simulink model "FireFighter_original"  (R2014a)
settings: Solver=ode45  StartTime=0.0  StopTime=150  RelTol=1e-3
undefined symbols (not defined in the file): DiscIntNeverNeededParam, sigbuilder_block
libraries: simulink x68
(part 6 of 6)

== system FireFighter_original/FF_Signals4/Inaccuracy2/Subsystem2/FireFighter ==
  note: current speed
  note: speed=90
  pos : Inport
  Constant : Constant  Value=0
  Constant1 : Constant  Value=0
  Constant2 : Constant  Value=0
  Discrete Derivative : simulink/Discrete/Discrete Derivative  gainval=1.0  ICPrevScaledInput=0.0  InputProcessing=Inherited  OutMin=[]  OutMax=[]  OutDataType=fixdt(1, 16)  OutScaling=2^-10  DoSatur=off
  Discrete PID Controller : simulink/Continuous/PID Controller  Controller=PI  TimeDomain=Discrete-time  SampleTime=-1  IntegratorMethod=Forward Euler  FilterMethod=Forward Euler  Form=Parallel  P=0.05  I=0.000228325  D=0  N=100  InitialConditionSource=internal  InitialConditionForIntegrator=0  InitialConditionForFilter=0  ExternalReset=none  LimitOutput=on  UpperSaturationLimit=1  LowerSaturationLimit=-1  LinearizeAsGain=off  AntiWindupMode=back-calculation  Kb=0.01  TrackingMode=off  Kt=1  PParamMin=[]  PParamMax=[]  IParamMin=[]  IParamMax=[]  DParamMin=[]  DParamMax=[]  NParamMin=[]  NParamMax=[]  KbParamMin=[]  KbParamMax=[]  KtParamMin=[]  KtParamMax=[]  POutMin=[]  POutMax=[]  IOutMin=[]  IOutMax=[]  DOutMin=[]  DOutMax=[]  NOutMin=[]  NOutMax=[]  KbOutMin=[]  KbOutMax=[]  KtOutMin=[]  KtOutMax=[]  IntegratorOutMin=[]  IntegratorOutMax=[]  FilterOutMin=[]  FilterOutMax=[]  SumOutMin=[]  SumOutMax=[]  SumI1OutMin=[]  SumI1OutMax=[]  SumI2OutMin=[]  SumI2OutMax=[]  SumI3OutMin=[]  SumI3OutMax=[]  SumDOutMin=[]  SumDOutMax=[]  SaturationOutMin=[]  SaturationOutMax=[]  IntegratorContinuousStateAttributes=''  IntegratorStateMustResolveToSignalObject=off  IntegratorRTWStateStorageClass=Auto  FilterContinuousStateAttributes=''  FilterStateMustResolveToSignalObject=off  FilterRTWStateStorageClass=Auto
  Discrete PID Controller1 : simulink/Continuous/PID Controller  Controller=PI  TimeDomain=Discrete-time  SampleTime=-1  IntegratorMethod=Forward Euler  FilterMethod=Forward Euler  Form=Parallel  P=0.05  I=0.000228325  D=0  N=100  InitialConditionSource=internal  InitialConditionForIntegrator=0  InitialConditionForFilter=0  ExternalReset=none  LimitOutput=on  UpperSaturationLimit=1  LowerSaturationLimit=-1  LinearizeAsGain=off  AntiWindupMode=back-calculation  Kb=0.01  TrackingMode=off  Kt=1  PParamMin=[]  PParamMax=[]  IParamMin=[]  IParamMax=[]  DParamMin=[]  DParamMax=[]  NParamMin=[]  NParamMax=[]  KbParamMin=[]  KbParamMax=[]  KtParamMin=[]  KtParamMax=[]  POutMin=[]  POutMax=[]  IOutMin=[]  IOutMax=[]  DOutMin=[]  DOutMax=[]  NOutMin=[]  NOutMax=[]  KbOutMin=[]  KbOutMax=[]  KtOutMin=[]  KtOutMax=[]  IntegratorOutMin=[]  IntegratorOutMax=[]  FilterOutMin=[]  FilterOutMax=[]  SumOutMin=[]  SumOutMax=[]  SumI1OutMin=[]  SumI1OutMax=[]  SumI2OutMin=[]  SumI2OutMax=[]  SumI3OutMin=[]  SumI3OutMax=[]  SumDOutMin=[]  SumDOutMax=[]  SaturationOutMin=[]  SaturationOutMax=[]  IntegratorContinuousStateAttributes=''  IntegratorStateMustResolveToSignalObject=off  IntegratorRTWStateStorageClass=Auto  FilterContinuousStateAttributes=''  FilterStateMustResolveToSignalObject=off  FilterRTWStateStorageClass=Auto
  Fast - to -Slow : RateTransition  OutPortSampleTimeMultiple=0.05  OutPortSampleTime=0.1
  Fast - to -Slow1 : RateTransition  OutPortSampleTimeMultiple=0.05  OutPortSampleTime=0.1
  Fast - to -Slow2 : RateTransition  OutPortSampleTimeMultiple=0.05  OutPortSampleTime=0.1
  Gain1 : Gain  Gain=-1
  Scope{1..2,4..9,11..13} (11 alike) : Scope
      Scope1 settings: YMin=-300  YMax=300  SaveName=ScopeData52
      Scope11 settings: YMin=-300  YMax=300  SaveName=ScopeData28
      Scope12 settings: YMin=-300  YMax=300  SaveName=ScopeData30
      Scope13 settings: SaveName=ScopeData31
      Scope2 settings: YMin=-300  YMax=300  SaveName=ScopeData2
      Scope4 settings: YMin=-300  YMax=300  SaveName=ScopeData17
      Scope5 settings: SaveName=ScopeData20
      Scope6 settings: YMin=-300  YMax=300  SaveName=ScopeData18
      Scope7 settings: YMin=-300  YMax=300  SaveName=ScopeData24
      Scope8 settings: TimeRange=10  SaveName=ScopeData25
      Scope9 settings: SaveName=ScopeData38
  Slow - to - Fast : RateTransition  OutPortSampleTimeMultiple=0.05  OutPortSampleTime=0.05
  Slow - to - Fast1 : RateTransition  OutPortSampleTimeMultiple=0.05  OutPortSampleTime=0.05
  Sum : Sum  Inputs=|+-
  Switch : Switch
  Switch1 : Switch
  gas : Outport
  brake : Outport  Port=2
  wires:
  Discrete Derivative/1 -> Scope8/1, Sum/2
  Discrete PID Controller/1 -> Scope2/1, Scope7/1, Switch/1, Switch/2, Switch1/2, Gain1/1
  Gain1/1 -> Switch1/3
  Switch/1 -> Slow - to - Fast/1, Scope4/1
  Constant/1 -> Switch/3, Switch1/1
  Switch1/1 -> Slow - to - Fast1/1, Scope6/1
  pos/1 -> Scope13/1, Fast - to -Slow/1
  Sum/1 -> Discrete PID Controller/1, Scope9/1
  Fast - to -Slow/1 -> Discrete Derivative/1, Scope5/1
  Slow - to - Fast/1 -> Scope11/1, gas/1
  Slow - to - Fast1/1 -> Scope12/1, brake/1
  Constant2/1 -> Fast - to -Slow1/1
  Fast - to -Slow1/1 -> Sum/1
  Discrete PID Controller1/1 -> Scope1/1
  Constant1/1 -> Fast - to -Slow2/1
  Fast - to -Slow2/1 -> Discrete PID Controller1/1

== stateflow chart FireFighter_original/Helicopter1 ==
  state FlyOn
    en:
    hold = 1;
    during:
    HFFPos = FFPos;
    HPos = HPos_In;
    inacc = FFPosInacc[1] - FFPosInacc[0];
    Signal_Reply_Out[0] =Signal_In[0];
    Signal_Reply_Out[1] =Signal_In[1];
    state srchID=getClosest [function]
      state [min,max] = getComposedInaccuracy(min1,max1, min2,max2) [function]
        state x_abs =abs(x) [function]
          (default) -> (junction 3808)
          (junction 3808) -> (junction 3809) [order 1] : [x < 0]
          (junction 3808) -> (junction 3810) [order 2] : {x_abs = x;}
          (junction 3809) -> (junction 3811) : {x_abs = -1*x;}
          (junction 3811) -> (junction 3810)
          (junction 3810) -> (junction 3812)
        (default) -> (junction 3780)
        (junction 3780) -> (junction 3785) : {val[0] = abs(min2 - min1);
            | val[1] = abs(max2 - min1);
            | val[2] = abs(min2 - max1);
            | val[3] = abs(max2 - max1);
            | min = val[0];
            | max = val[0];
            | j =1;}
        (junction 3781) -> (junction 3782) [order 1] : [min > val[j]]
        (junction 3785) -> (junction 3781) [order 1] : [j<4]
        (junction 3781) -> (junction 3783) [order 2]
        (junction 3782) -> (junction 3784) : {min = val[j];}
        (junction 3784) -> (junction 3783)
        (junction 3783) -> (junction 3786)
        (junction 3789) -> (junction 3785) : {j++;}
        (junction 3785) -> (junction 3788) [order 2]
        (junction 3786) -> (junction 3787) [order 1] : [max < val[j]]
        (junction 3787) -> (junction 3790) : {max = val[j];}
        (junction 3786) -> (junction 3789) [order 2]
        (junction 3790) -> (junction 3789)
      (default) -> (junction 3745)
      (junction 3745) -> (junction 3746) : {
          | [Min[0],Max[0]]=getComposedInaccuracy(FFPosInacc[0],FFPosInacc[1],FFPos,FFPos);
          | [Min[1],Max[1]]=getComposedInaccuracy(FFPosInacc[0],FFPosInacc[1],HsPosInacc[0],HsPosInacc[1]);
          | [Min[2],Max[2]]=getComposedInaccuracy(FFPosInacc[0],FFPosInacc[1],HsPosInacc[2],HsPosInacc[3]);
          | inacc_min = Min[0];
          | srchID = HID;
          | i =1;
          | }
      (junction 3736) -> (junction 3724) [order 1] : [inacc_min > Min[i]]
      (junction 3746) -> (junction 3736) [order 1] : [i<3]
      (junction 3736) -> (junction 3738) [order 2]
      (junction 3724) -> (junction 3732) : {inacc_min = Min[i]; srchID = OHIDs[i-1];}
      (junction 3738) -> (junction 3746) : {i++;}
      (junction 3746) -> (junction 3740) [order 2]
      (junction 3732) -> (junction 3738)
    state inaccFuture=getInacc(dt) [function]
      (default) -> (junction 3488)
      (junction 3488) -> (junction 3489) [order 1] : [true]
      (junction 3488) -> (junction 3490) [order 2]
      (junction 3489) -> (junction 3491) : {inaccFuture = dt*inacc;}
      (junction 3491) -> (junction 3490)
      (junction 3490) -> (junction 3492)
    state Mediate
      en:
      time_last =0;
      time_period = 0;
      time_val = temporalCount(sec);
      du:
      time_val = temporalCount(sec);
    state HsSignals [function]
      (default) -> (junction 3581)
      (junction 3581) -> (junction 3580) [order 1] : [(Signal_Reply_In[0] != Signal_Out || Signal_Reply_In[0] != Signal_Out) && time_period < (time_val - time_last)]
      (junction 3581) -> (junction 3583) [order 2]
      (junction 3580) -> (junction 3586) : {time_period = time_val - time_last;}
      (junction 3583) -> (junction 3582) [order 1] : [Signal_Reply_In[0] == Signal_Out &&Signal_Reply_In[1] == Signal_Out]
      (junction 3583) -> (junction 3584) [order 2]
      (junction 3582) -> (junction 3585) : {Signal_Out = time_val; time_last = Signal_Out; }
      (junction 3585) -> (junction 3584)
      (junction 3586) -> (junction 3585)
      (junction 3584) -> (junction 3587)
    state OrganizeSearch
      en:
      hold = 0;
      time_last =0;
      time_period = 0;
      time_val = temporalCount(sec);
      Signal_Out = time_val;
      SearchID = getClosest();
      du:
      HsSignals();
      SearchID = getClosest();
      time_val = temporalCount(sec);
      ex:
      hold = 1;
      state InitializedSearch
      state LeadSearch
      state OtherSearch
        du:
        Search_Out = SearchID;
        ex:
        Search_Out = 0;
      (default) -> InitializedSearch
      InitializedSearch -> LeadSearch [order 1] : [SearchID == HID]
      InitializedSearch -> OtherSearch [order 2] : [SearchID != HID]
      OtherSearch -> LeadSearch : [SearchID == HID]
      LeadSearch -> OtherSearch : [SearchID != HID]
    state ToldToSearch
      en: hold = 0;
      ex: hold = 1;
    state InitializedSystem
      en:
      hold = 0;
      HFFPos = 0;
      ex:
      hold = 1;
    InitializedSystem -> Mediate [order 1] : [MID == HID]
    Mediate -> InitializedSystem [order 2] : [MID != HID && MID !=0]
    OrganizeSearch -> Mediate [order 1] : [inacc <= 5000]
    Mediate -> OrganizeSearch [order 1] : [ inacc > 5000  ]
    InitializedSystem -> ToldToSearch [order 2] : [Search_In[0] == HID || Search_In[1] == HID]
    ToldToSearch -> InitializedSystem : [Search_In[0] != HID && Search_In[1] != HID]
    (default) -> InitializedSystem
    OrganizeSearch -> InitializedSystem [order 2] : [MID != HID && MID !=0]
    OrganizeSearch -> InitializedSystem [order 3] : [(inacc+getInacc(time_period))  > 10000]
  state FlyOff
  FlyOn -> FlyOff : [SWITCH==0]
  FlyOff -> FlyOn : [SWITCH==1]
  (default) -> FlyOff
  data: x function_input double; x_abs function_output double; min1 function_input double; max1 function_input double; min function_output double; max function_output double; val temporary double size=4; min2 function_input double; max2 function_input double; j local double; srchID function_output double; Max temporary double size=3; Min temporary double size=3; inacc1 temporary double size=2; i local double; inacc_min local double; inaccFuture function_output double; dt function_input double; HID output =1; FFPos input; HFFPos output; HPos output double =0; HPos_In input double; FFPosInacc input size=2; HsPosInacc input size=4; SWITCH input double; OHIDs input size=2; OHPoss input size=2; OHFFPos input size=2; Search_In input size=2; SearchID local double; Search_Loc local double; MID input; Signal_In input size=2; Signal_Out output; Search_Out output; time_val local double; Signal_Reply_Out output size=2; Signal_Reply_In input size=2; valFF local double; time_period local double; time_last local double; inacc local double; hold output double

== stateflow chart FireFighter_original/Helicopter2 ==
  state FlyOn
    en:
    hold = 1;
    during:
    HFFPos = FFPos;
    HPos = HPos_In;
    inacc = FFPosInacc[1] - FFPosInacc[0];
    Signal_Reply_Out[0] =Signal_In[0];
    Signal_Reply_Out[1] =Signal_In[1];
    state srchID=getClosest [function]
      state [min,max] = getComposedInaccuracy(min1,max1, min2,max2) [function]
        state x_abs =abs(x) [function]
          (default) -> (junction 3883)
          (junction 3883) -> (junction 3884) [order 1] : [x < 0]
          (junction 3883) -> (junction 3885) [order 2] : {x_abs = x;}
          (junction 3884) -> (junction 3886) : {x_abs = -1*x;}
          (junction 3886) -> (junction 3885)
          (junction 3885) -> (junction 3887)
        (default) -> (junction 3855)
        (junction 3855) -> (junction 3860) : {val[0] = abs(min2 - min1);
            | val[1] = abs(max2 - min1);
            | val[2] = abs(min2 - max1);
            | val[3] = abs(max2 - max1);
            | min = val[0];
            | max = val[0];
            | j =1;}
        (junction 3856) -> (junction 3857) [order 1] : [min > val[j]]
        (junction 3860) -> (junction 3856) [order 1] : [j<4]
        (junction 3856) -> (junction 3858) [order 2]
        (junction 3857) -> (junction 3859) : {min = val[j];}
        (junction 3859) -> (junction 3858)
        (junction 3858) -> (junction 3861)
        (junction 3864) -> (junction 3860) : {j++;}
        (junction 3860) -> (junction 3863) [order 2]
        (junction 3861) -> (junction 3862) [order 1] : [max < val[j]]
        (junction 3862) -> (junction 3865) : {max = val[j];}
        (junction 3861) -> (junction 3864) [order 2]
        (junction 3865) -> (junction 3864)
      (default) -> (junction 3830)
      (junction 3830) -> (junction 3833) : {
          | [Min[0],Max[0]]=getComposedInaccuracy(FFPosInacc[0],FFPosInacc[1],FFPos,FFPos);
          | [Min[1],Max[1]]=getComposedInaccuracy(FFPosInacc[0],FFPosInacc[1],HsPosInacc[0],HsPosInacc[1]);
          | [Min[2],Max[2]]=getComposedInaccuracy(FFPosInacc[0],FFPosInacc[1],HsPosInacc[2],HsPosInacc[3]);
          | inacc_min = Min[0];
          | srchID = HID;
          | i =1;
          | }
      (junction 3831) -> (junction 3832) [order 1] : [inacc_min > Min[i]]
      (junction 3833) -> (junction 3831) [order 1] : [i<3]
      (junction 3831) -> (junction 3834) [order 2]
      (junction 3832) -> (junction 3835) : {inacc_min = Min[i]; srchID = OHIDs[i-1];}
      (junction 3834) -> (junction 3833) : {i++;}
      (junction 3833) -> (junction 3836) [order 2]
      (junction 3835) -> (junction 3834)
    state inaccFuture=getInacc(dt) [function]
      (default) -> (junction 3488)
      (junction 3488) -> (junction 3489) [order 1] : [true]
      (junction 3488) -> (junction 3490) [order 2]
      (junction 3489) -> (junction 3491) : {inaccFuture = dt*inacc;}
      (junction 3491) -> (junction 3490)
      (junction 3490) -> (junction 3492)
    state Mediate
      en:
      time_last =0;
      time_period = 0;
      time_val = temporalCount(sec);
      du:
      time_val = temporalCount(sec);
    state HsSignals [function]
      (default) -> (junction 3581)
      (junction 3581) -> (junction 3580) [order 1] : [(Signal_Reply_In[0] != Signal_Out || Signal_Reply_In[0] != Signal_Out) && time_period < (time_val - time_last)]
      (junction 3581) -> (junction 3583) [order 2]
      (junction 3580) -> (junction 3586) : {time_period = time_val - time_last;}
      (junction 3583) -> (junction 3582) [order 1] : [Signal_Reply_In[0] == Signal_Out &&Signal_Reply_In[1] == Signal_Out]
      (junction 3583) -> (junction 3584) [order 2]
      (junction 3582) -> (junction 3585) : {Signal_Out = time_val; time_last = Signal_Out; }
      (junction 3585) -> (junction 3584)
      (junction 3586) -> (junction 3585)
      (junction 3584) -> (junction 3587)
    state OrganizeSearch
      en:
      hold = 0;
      time_last =0;
      time_period = 0;
      time_val = temporalCount(sec);
      Signal_Out = time_val;
      SearchID = getClosest();
      du:
      HsSignals();
      SearchID = getClosest();
      time_val = temporalCount(sec);
      ex:
      hold = 1;
      state InitializeSearch
      state LeadSearch
      state OtherSearch
        du:
        Search_Out = SearchID;
        ex:
        Search_Out = 0;
      (default) -> InitializeSearch
      InitializeSearch -> LeadSearch [order 1] : [SearchID == HID]
      InitializeSearch -> OtherSearch [order 2] : [SearchID != HID]
      OtherSearch -> LeadSearch : [SearchID == HID]
      LeadSearch -> OtherSearch : [SearchID != HID]
    state ToldToSearch
      en: hold = 0;
      ex: hold = 1;
    state InitializedSystem
      en:
      hold = 0;
      HFFPos = 0;
      ex:
      hold = 1;
    InitializedSystem -> Mediate [order 1] : [MID == HID]
    Mediate -> InitializedSystem [order 2] : [MID != HID && MID !=0]
    OrganizeSearch -> Mediate [order 1] : [inacc <= 5000]
    Mediate -> OrganizeSearch [order 1] : [ inacc > 5000  ]
    InitializedSystem -> ToldToSearch [order 2] : [Search_In[0] == HID || Search_In[1] == HID]
    ToldToSearch -> InitializedSystem : [Search_In[0] != HID && Search_In[1] != HID]
    (default) -> InitializedSystem
    OrganizeSearch -> InitializedSystem [order 2] : [MID != HID && MID !=0]
    OrganizeSearch -> InitializedSystem [order 3] : [(inacc+getInacc(time_period))  > 10000]
  state FlyOff
  FlyOn -> FlyOff : [SWITCH==0]
  FlyOff -> FlyOn : [SWITCH==1]
  (default) -> FlyOff
  data: x function_input double; x_abs function_output double; min1 function_input double; max1 function_input double; min function_output double; max function_output double; val temporary double size=4; min2 function_input double; max2 function_input double; j local double; srchID function_output double; Max temporary double size=3; Min temporary double size=3; inacc1 temporary double size=2; i local double; inacc_min local double; inaccFuture function_output double; dt function_input double; HID output =2; FFPos input; HFFPos output; HPos output double =0; HPos_In input double; FFPosInacc input size=2; HsPosInacc input size=4; SWITCH input double; OHIDs input size=2; OHPoss input size=2; OHFFPos input size=2; Search_In input size=2; SearchID local double; Search_Loc local double; MID input; Signal_In input size=2; Signal_Out output; Search_Out output; time_val local double; Signal_Reply_Out output size=2; Signal_Reply_In input size=2; valFF local double; time_period local double; time_last local double; inacc local double; hold output double

== stateflow chart FireFighter_original/Helicopter3 ==
  state FlyOn
    en:
    hold = 1;
    during:
    HFFPos = FFPos;
    HPos = HPos_In;
    inacc = FFPosInacc[1] - FFPosInacc[0];
    Signal_Reply_Out[0] =Signal_In[0];
    Signal_Reply_Out[1] =Signal_In[1];
    state srchID=getClosest [function]
      state [min,max] = getComposedInaccuracy(min1,max1, min2,max2) [function]
        state x_abs =abs(x) [function]
          (default) -> (junction 3883)
          (junction 3883) -> (junction 3884) [order 1] : [x < 0]
          (junction 3883) -> (junction 3885) [order 2] : {x_abs = x;}
          (junction 3884) -> (junction 3886) : {x_abs = -1*x;}
          (junction 3886) -> (junction 3885)
          (junction 3885) -> (junction 3887)
        (default) -> (junction 3855)
        (junction 3855) -> (junction 3860) : {val[0] = abs(min2 - min1);
            | val[1] = abs(max2 - min1);
            | val[2] = abs(min2 - max1);
            | val[3] = abs(max2 - max1);
            | min = val[0];
            | max = val[0];
            | j =1;}
        (junction 3856) -> (junction 3857) [order 1] : [min > val[j]]
        (junction 3860) -> (junction 3856) [order 1] : [j<4]
        (junction 3856) -> (junction 3858) [order 2]
        (junction 3857) -> (junction 3859) : {min = val[j];}
        (junction 3859) -> (junction 3858)
        (junction 3858) -> (junction 3861)
        (junction 3864) -> (junction 3860) : {j++;}
        (junction 3860) -> (junction 3863) [order 2]
        (junction 3861) -> (junction 3862) [order 1] : [max < val[j]]
        (junction 3862) -> (junction 3865) : {max = val[j];}
        (junction 3861) -> (junction 3864) [order 2]
        (junction 3865) -> (junction 3864)
      (default) -> (junction 3830)
      (junction 3830) -> (junction 3833) : {
          | [Min[0],Max[0]]=getComposedInaccuracy(FFPosInacc[0],FFPosInacc[1],FFPos,FFPos);
          | [Min[1],Max[1]]=getComposedInaccuracy(FFPosInacc[0],FFPosInacc[1],HsPosInacc[0],HsPosInacc[1]);
          | [Min[2],Max[2]]=getComposedInaccuracy(FFPosInacc[0],FFPosInacc[1],HsPosInacc[2],HsPosInacc[3]);
          | inacc_min = Min[0];
          | srchID = HID;
          | i =1;
          | }
      (junction 3831) -> (junction 3832) [order 1] : [inacc_min > Min[i]]
      (junction 3833) -> (junction 3831) [order 1] : [i<3]
      (junction 3831) -> (junction 3834) [order 2]
      (junction 3832) -> (junction 3835) : {inacc_min = Min[i]; srchID = OHIDs[i-1];}
      (junction 3834) -> (junction 3833) : {i++;}
      (junction 3833) -> (junction 3836) [order 2]
      (junction 3835) -> (junction 3834)
    state inaccFuture=getInacc(dt) [function]
      (default) -> (junction 3488)
      (junction 3488) -> (junction 3489) [order 1] : [true]
      (junction 3488) -> (junction 3490) [order 2]
      (junction 3489) -> (junction 3491) : {inaccFuture = dt*inacc;}
      (junction 3491) -> (junction 3490)
      (junction 3490) -> (junction 3492)
    state Mediate
      en:
      time_last =0;
      time_period = 0;
      time_val = temporalCount(sec);
      du:
      time_val = temporalCount(sec);
    state HsSignals [function]
      (default) -> (junction 3581)
      (junction 3581) -> (junction 3580) [order 1] : [(Signal_Reply_In[0] != Signal_Out || Signal_Reply_In[0] != Signal_Out) && time_period < (time_val - time_last)]
      (junction 3581) -> (junction 3583) [order 2]
      (junction 3580) -> (junction 3586) : {time_period = time_val - time_last;}
      (junction 3583) -> (junction 3582) [order 1] : [Signal_Reply_In[0] == Signal_Out &&Signal_Reply_In[1] == Signal_Out]
      (junction 3583) -> (junction 3584) [order 2]
      (junction 3582) -> (junction 3585) : {Signal_Out = time_val; time_last = Signal_Out; }
      (junction 3585) -> (junction 3584)
      (junction 3586) -> (junction 3585)
      (junction 3584) -> (junction 3587)
    state OrganizeSearch
      en:
      hold = 0;
      time_last =0;
      time_period = 0;
      time_val = temporalCount(sec);
      Signal_Out = time_val;
      SearchID = getClosest();
      du:
      HsSignals();
      SearchID = getClosest();
      time_val = temporalCount(sec);
      ex:
      hold = 1;
      state InitializeSearch
      state LeadSearch
      state OtherSearch
        du:
        Search_Out = SearchID;
        ex:
        Search_Out = 0;
      (default) -> InitializeSearch
      InitializeSearch -> LeadSearch [order 1] : [SearchID == HID]
      InitializeSearch -> OtherSearch [order 2] : [SearchID != HID]
      OtherSearch -> LeadSearch : [SearchID == HID]
      LeadSearch -> OtherSearch : [SearchID != HID]
    state ToldToSearch
      en: hold = 0;
      ex: hold = 1;
    state InitializedSystem
      en:
      hold = 0;
      HFFPos = 0;
      ex:
      hold = 1;
    InitializedSystem -> Mediate [order 1] : [MID == HID]
    Mediate -> InitializedSystem [order 2] : [MID != HID && MID !=0]
    OrganizeSearch -> Mediate [order 1] : [inacc <= 5000]
    Mediate -> OrganizeSearch [order 1] : [ inacc > 5000 ]
    InitializedSystem -> ToldToSearch [order 2] : [Search_In[0] == HID || Search_In[1] == HID]
    ToldToSearch -> InitializedSystem : [Search_In[0] != HID && Search_In[1] != HID]
    (default) -> InitializedSystem
    OrganizeSearch -> InitializedSystem [order 2] : [MID != HID && MID !=0]
    OrganizeSearch -> InitializedSystem [order 3] : [(inacc+getInacc(time_period))  > 10000]
  state FlyOff
  FlyOn -> FlyOff : [SWITCH==0]
  FlyOff -> FlyOn : [SWITCH==1]
  (default) -> FlyOff
  data: x function_input double; x_abs function_output double; min1 function_input double; max1 function_input double; min function_output double; max function_output double; val temporary double size=4; min2 function_input double; max2 function_input double; j local double; srchID function_output double; Max temporary double size=3; Min temporary double size=3; inacc1 temporary double size=2; i local double; inacc_min local double; inaccFuture function_output double; dt function_input double; HID output =3; FFPos input; HFFPos output; HPos output double =0; HPos_In input double; FFPosInacc input size=2; HsPosInacc input size=4; SWITCH input double; OHIDs input size=2; OHPoss input size=2; OHFFPos input size=2; Search_In input size=2; SearchID local double; Search_Loc local double; MID input; Signal_In input size=2; Signal_Out output; Search_Out output; time_val local double; Signal_Reply_Out output size=2; Signal_Reply_In input size=2; valFF local double; time_period local double; time_last local double; inacc local double; hold output double

== stateflow chart FireFighter_original/Leader ==
  state LeaderLogic
    du:
    FFPos = FFPos_In;
    inacc = FFPosInacc[1] - FFPosInacc[0];
    state InitilizedLeader
    state FFConnected
    state Alarmed
    (default) -> InitilizedLeader
    InitilizedLeader -> FFConnected [order 1] : [inacc <= 10000]
    InitilizedLeader -> Alarmed [order 2] : [inacc > 10000]
    FFConnected -> Alarmed : [inacc > 10000]
    Alarmed -> FFConnected : [inacc <= 10000]
  data: FFPos_In input; FFPosInacc input size=2; HFFPoss input size=3; HIDs input size=3; HPoss input size=3; FFPos local double; inacc_val local double; counter local double; inacc_max local double; inacc_min local double; inacc local double

== stateflow chart FireFighter_original/FireFighter ==
  state Active
    en:
    ffPos = 0;
    ffHold = 1;
    during:
    ffPos = ffPos_In;
    state Wait
    state LeaderConnected
      en:
      ffHold = 0;
      ex:
      ffHold = 1;
    state MediatorConnected
      en:
      ffMID=0;
      ffHold = 0;
      du:
      MIDValue();
      ex:
      ffMID=0;
      ffHold = 1;
    (default) -> Wait
    Wait -> LeaderConnected [order 1] : [ffConn > 0]
    Wait -> MediatorConnected [order 2] : [ffHconn[0] > 0 || ffHconn[1] > 0 || ffHconn[2] > 0]
    LeaderConnected -> Wait : [ffConn == 0]
    MediatorConnected -> Wait : [ffHconn[0] == 0 && ffHconn[1] == 0 && ffHconn[2] == 0]
  state MIDValue [function]
    (default) -> (junction 1709) : /* write the MID */
    (junction 1709) -> (junction 1711) [order 1] : [ffHconn[0] > 0]
    (junction 1709) -> (junction 1710) [order 2]
    (junction 1711) -> (junction 1716) : {ffMID = 1;}
    (junction 1710) -> (junction 1715) [order 1] : [ffHconn[1] > 0]
    (junction 1710) -> (junction 1717) [order 2]
    (junction 1715) -> (junction 1712) : {ffMID = 2;}
    (junction 1717) -> (junction 1718) [order 1] : [ffHconn[2] > 0]
    (junction 1717) -> (junction 1713) [order 2] : {ffMID = 0;}
    (junction 1718) -> (junction 1719) : {ffMID = 3;}
    (junction 1719) -> (junction 1713)
    (junction 1712) -> (junction 1719)
    (junction 1716) -> (junction 1712)
    (junction 1713) -> (junction 1714)
  state Inactive
  Inactive -> Active : [ffActivate==1]
  Active -> Inactive : [ffActivate==0]
  (default) -> Inactive
  data: ffConn input; ffHconn input size=3; ffPos output double; ffPos_In input; ffMID output; ffActivate input double; ffHold output double
